simulink model "HH_Neuron"  (R2022b)
settings: Solver=VariableStepAuto  StartTime=0.0  StopTime=600e-3  RelTol=1e-3
settings Model: Creator=Serious Chimp  LastModifiedBy=Serious Chimp
settings OptimizationCC: ReuseModelBlockBuffer=on

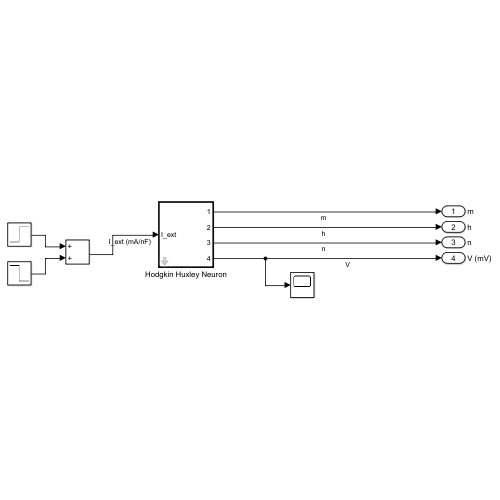
[thumbnail: Simulink's stored preview of the top-level diagram]
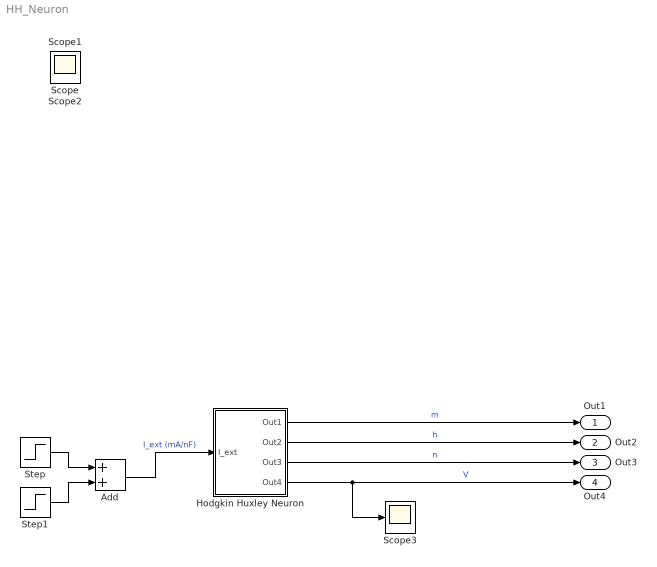
== system HH_Neuron ==
  Add : Sum
  Hodgkin Huxley Neuron : Subsystem  TreatAsAtomicUnit=on  mask{g_Na=120, e_Na=115, g_K=36, e_K=-12, g_L=0.3, e_L=10.6, m0=0.1, h0=0.6, n0=0.31, V0=0}
      mask prompts: g_Na "Sodium Conductance, g_Na"; e_Na "Sodium Eqm Voltage, e_Na"; g_K "Potassium Conductance, g_K"; e_K "Potassium Eqm Votlage, e_K"; g_L "Leakage Conductance, g_L"; e_L "Leakage Eqm Votlage, e_L"; m0 "Initial, m0"; h0 "Initial, h0"; n0 "Initial, n0"; V0 "Equilibrium, V0"
  Scope{,1..3} (4 alike) : Scope
  Step : Step  Time=250e-3  After=4  SampleTime=0
  Step1 : Step  Time=350e-3  After=-4  SampleTime=0
  Out1 : Outport  SignalName=m
  Out2 : Outport  Port=2  SignalName=h
  Out3 : Outport  Port=3  SignalName=n
  Out4 : Outport  Port=4  SignalName=V (mV)
  wires:
  Hodgkin Huxley Neuron/1(Out1) -> Out1/1  "m"
  Hodgkin Huxley Neuron/2(Out2) -> Out2/1  "h"
  Hodgkin Huxley Neuron/3(Out3) -> Out3/1  "n"
  Hodgkin Huxley Neuron/4(Out4) -> Scope3/1, Out4/1  "V"
  Step/1 -> Add/1
  Step1/1 -> Add/2
  Add/1 -> Hodgkin Huxley Neuron/1(I_ext)  "I_ext (mA/nF)"

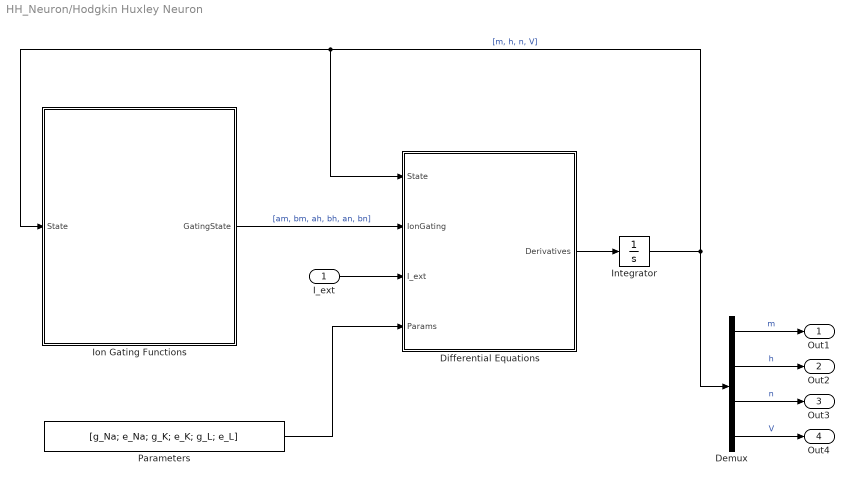
== system HH_Neuron/Hodgkin Huxley Neuron ==
  I_ext : Inport
  Demux : Demux
  Differential Equations : MATLAB Function  TreatAsAtomicUnit=on
  Integrator : Integrator  InitialCondition=[m0 h0 n0 V0]
  Ion Gating Functions : MATLAB Function  TreatAsAtomicUnit=on
  Parameters : Constant  Value=[g_Na; e_Na; g_K; e_K; g_L; e_L]
  Out1 : Outport
  Out2 : Outport  Port=2
  Out3 : Outport  Port=3
  Out4 : Outport  Port=4
  wires:
  Demux/3 -> Out3/1  "n"
  Demux/4 -> Out4/1  "V"
  Ion Gating Functions/1(GatingState) -> Differential Equations/2(IonGating)  "[am, bm, ah, bh, an, bn]"
  I_ext/1 -> Differential Equations/3(I_ext)
  Integrator/1 -> Ion Gating Functions/1(State), Differential Equations/1(State), Demux/1  "[m, h, n, V]"
  Parameters/1 -> Differential Equations/4(Params)
  Demux/1 -> Out1/1  "m"
  Demux/2 -> Out2/1  "h"
  Differential Equations/1(Derivatives) -> Integrator/1

== matlab function HH_Neuron/Hodgkin Huxley Neuron/Differential Equations ==
  data: State input; IonGating input; I_ext input; Derivatives output; Params input
function Derivatives = ODE(State, IonGating, I_ext, Params)
    am = IonGating(1);
    bm = IonGating(2);
    ah = IonGating(3);
    bh = IonGating(4);
    an = IonGating(5);
    bn = IonGating(6);

    m = State(1);
    h = State(2);
    n = State(3);
    v = State(4);

    g_Na = Params(1);  
    e_Na = Params(2);  
    g_K = Params(3);   
    e_K = Params(4);  
    g_L = Params(5);      
    e_L = Params(6);  

    m_dot = 1000*(am*(1-m) - bm*m);
    h_dot = 1000*(ah*(1-h) - bh*h);
    n_dot = 1000*(an*(1-n) - bn*n);

    v_dot = 1000*(-(g_Na * m^3 * h * (v - e_Na)) - (g_K * n^4 * (v - e_K)) - (g_L * (v - e_L)) + I_ext);

    Derivatives = [m_dot, h_dot, n_dot, v_dot];

end

== matlab function HH_Neuron/Hodgkin Huxley Neuron/Ion Gating Functions ==
  data: State input; GatingState output
function GatingState = AlphaBeta(State)

V = State(4);

am = (2.5-0.1*V) / (exp(2.5-0.1*V) -1);
bm = 4*exp(-V/18);
ah = 0.07*exp(-V/20);
bh = 1/(exp(3.0-0.1*V)+1);
an = (0.1-0.01*V) / (exp(1-0.1*V) -1);
bn = 0.125*exp(-V/80);

GatingState = [am, bm, ah, bh, an, bn];
end
